simulink model "quat2att"  (R2018a)
settings: Solver=VariableStepAuto  StartTime=0.0  StopTime=10.0  RelTol=1e-3
settings Model: Creator=lamy  LastModifiedBy=lamy

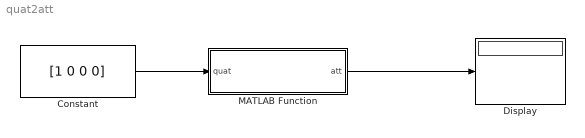
== system quat2att ==
  Constant : Constant  Value=[1 0 0 0]  VectorParams1D=off
  Display : Display
  MATLAB Function : MATLAB Function  TreatAsAtomicUnit=on
  wires:
  Constant/1 -> MATLAB Function/1(quat)
  MATLAB Function/1(att) -> Display/1

== matlab function quat2att/MATLAB Function ==
  data: quat input; att output
function att = quat2att(quat)
yaw = atan2(2*(quat(1)*quat(4) + quat(2)*quat(3)), 1-2*(quat(3)^2 + quat(4)^2));
pitch = asin(2*(quat(1)*quat(3) - quat(2)*quat(4)));
roll = atan2(2*(quat(1)*quat(2) + quat(3)*quat(4)), 1-2*(quat(2)^2 + quat(3)^2));
att = [roll; pitch; yaw];
